simulink model "Exercise11_3"
settings: Solver=ode45  SolverMode=SingleTasking  StartTime=0.0  StopTime=10.0  RelTol=1e-3
undefined symbols (not defined in the file or in its folder): f, J, ke, Kpot, kt, L, N, R
settings Model: Creator=Ramiro  LastModifiedBy=k340h17
settings DataIOCC: LimitDataPoints=on  SaveFormat=Array  SignalLoggingSaveFormat=ModelDataLogs  ReturnWorkspaceOutputs=off
settings OptimizationCC: BlockReduction=off  BooleanDataType=off  ExpressionDepthLimit=2147483647  LifeSpan=inf  SimCompilerOptimization=Off
settings DebuggingCC: SaveWithParameterizedLinksMsg=none  UnderspecifiedInitializationDetection=Classic  MergeDetectMultiDrivingBlocksExec=none  SignalResolutionControl=TryResolveAllWithWarning  MultiTaskDSMMsg=warning  MultiTaskCondExecSysMsg=none  FcnCallInpInsideContextMsg=Enable All  FrameProcessingCompatibilityMsg=warning  StateNameClashWarn=warning  StrictBusMsg=None  SFUnexpectedBacktrackingDiag=warning  SFNoUnconditionalDefaultTransitionDiag=warning
settings HardwareCC: ProdBitPerPointer=32  ProdLargestAtomicFloat=None  ProdIntDivRoundTo=Undefined  ProdEndianess=Unspecified  ProdWordSize=32  ProdHWDeviceType=32-bit Generic  TargetUnknown=on
settings ModelReferenceCC: PropagateSignalLabelsOutOfModel=off
settings SFSimCC: SimUseLocalCustomCode=off
settings RTWCC: RTWUseLocalCustomCode=off  IncludeERTFirstTime=on  RTWCompilerOptimization=Off
settings CodeAppCC: CustomSymbolStrType=$N$R$M
settings GRTTargetCC: CodeReplacementLibrary=ANSI_C  GeneratePreprocessorConditionals=Disable all  CPPClassGenCompliant=off

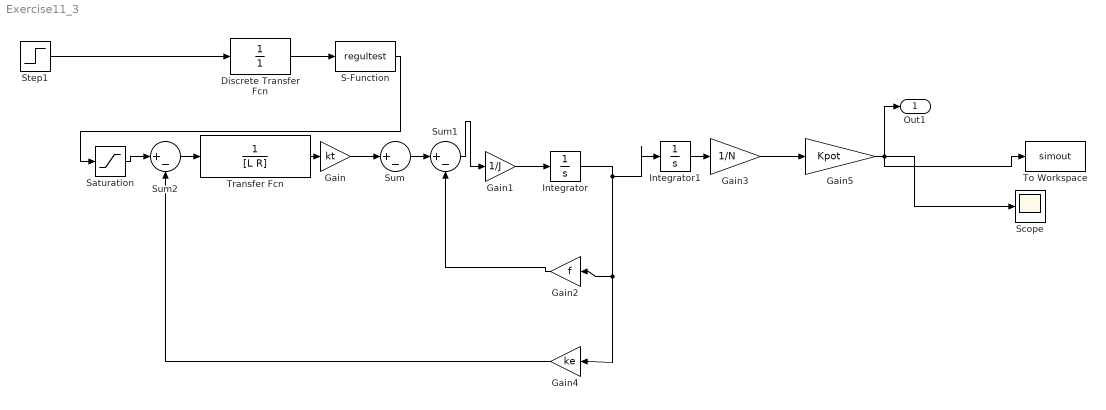
== system Exercise11_3 ==
  Discrete Transfer Fcn : DiscreteTransferFcn  Denominator=[1]  SampleTime=.00525
  Gain : Gain  Gain=kt
  Gain1 : Gain  Gain=1/J
  Gain2 : Gain  Gain=f
  Gain3 : Gain  Gain=1/N
  Gain4 : Gain  Gain=ke
  Gain5 : Gain  Gain=Kpot
  Integrator : Integrator
  Integrator1 : Integrator
  S-Function : S-Function  FunctionName=regultest  Parameters=85.96 -73.49 -0.4379  EnableBusSupport=off
  Saturation : Saturate  UpperLimit=10  LowerLimit=-10
  Scope : Scope
  Step1 : Step  SampleTime=0
  Sum : Sum  Inputs=|+-
  Sum1 : Sum  Inputs=|+-
  Sum2 : Sum  Inputs=|+-
  To Workspace : ToWorkspace  VariableName=simout  SampleTime=-1  SaveFormat=Structure With Time
  Transfer Fcn : TransferFcn  Denominator=[L R]
  Out1 : Outport
  wires:
  Sum/1 -> Sum1/1
  Sum1/1 -> Gain1/1
  Gain2/1 -> Sum1/2
  Transfer Fcn/1 -> Gain/1
  Sum2/1 -> Transfer Fcn/1
  Gain1/1 -> Integrator/1
  Integrator/1 -> Integrator1/1, Gain4/1, Gain2/1
  Gain5/1 -> Out1/1, Scope/1, To Workspace/1
  Gain3/1 -> Gain5/1
  Integrator1/1 -> Gain3/1
  Gain/1 -> Sum/1
  Gain4/1 -> Sum2/2
  Saturation/1 -> Sum2/1
  Step1/1 -> Discrete Transfer Fcn/1
  Discrete Transfer Fcn/1 -> S-Function/1
  S-Function/1 -> Saturation/1
